simulink model "test2"  (R2020a)
settings: Solver=VariableStepAuto  StartTime=0.0  StopTime=1000  RelTol=1e-3
undefined symbols (not defined in the file): Cb, Ch, Kb, Kh, Tout
libraries: simulink x2
settings Model: Creator=piyus  LastModifiedBy=piyus

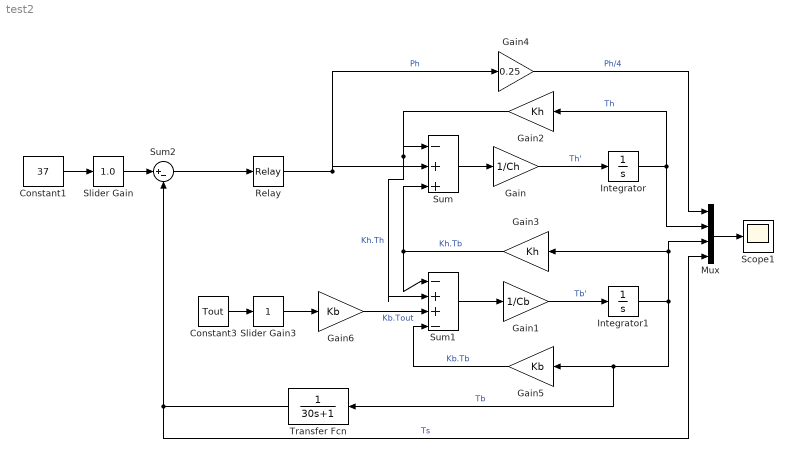
== system test2 ==
  Constant1 : Constant  Value=37  SampleTime=0.01
  Constant3 : Constant  Value=Tout
  Gain : Gain  Gain=1/Ch
  Gain1 : Gain  Gain=1/Cb
  Gain2 : Gain  Gain=Kh
  Gain3 : Gain  Gain=Kh
  Gain4 : Gain  Gain=0.25
  Gain5 : Gain  Gain=Kb
  Gain6 : Gain  Gain=Kb
  Integrator : Integrator  InitialCondition=25
  Integrator1 : Integrator  InitialCondition=25
  Mux : Mux
  Relay : Relay  OnSwitchValue=0.01/(0.19*2)+0.3  OffSwitchValue=-0.01/(0.19*2)+0.3  OnOutputValue=Ph
  Scope1 : Scope
  Slider Gain : simulink/Math Operations/Slider Gain  gain=1.0  low=0  high=1
  Slider Gain3 : simulink/Math Operations/Slider Gain  gain=1  low=0  high=2
  Sum : Sum  Inputs=|-++
  Sum1 : Sum  Inputs=|-++-
  Sum2 : Sum  Inputs=|+-
  Transfer Fcn : TransferFcn  Denominator=[30 1]
  wires:
  Integrator1/1 -> Gain5/1, Transfer Fcn/1, Mux/3, Gain3/1  "Tb"
  Integrator/1 -> Gain2/1, Mux/2  "Th"
  Mux/1 -> Scope1/1
  Gain/1 -> Integrator/1  "Th'"
  Sum/1 -> Gain/1
  Gain1/1 -> Integrator1/1  "Tb'"
  Sum1/1 -> Gain1/1
  Gain2/1 -> Sum1/2, Sum/1  "Kh.Th"
  Gain3/1 -> Sum/3, Sum1/1  "Kh.Tb"
  Constant3/1 -> Slider Gain3/1
  Relay/1 -> Gain4/1, Sum/2  "Ph"
  Slider Gain3/1 -> Gain6/1
  Gain5/1 -> Sum1/4  "Kb.Tb"
  Gain6/1 -> Sum1/3  "Kb.Tout"
  Gain4/1 -> Mux/1  "Ph/4"
  Constant1/1 -> Slider Gain/1
  Sum2/1 -> Relay/1
  Slider Gain/1 -> Sum2/1
  Transfer Fcn/1 -> Mux/4, Sum2/2  "Ts"
